simulink model "MCLV2_dsPIC33EP256MC506_externalOpAmp_DataLog"  (Simulink 9.2)
settings: Solver=FixedStepDiscrete  StartTime=0.0  StopTime=inf  FixedStep=.00005  RelTol=1e-3  EnableMultiTasking=on
undefined symbols (not defined in the file or in its folder): A4, A8, B5, B6, C10, C5, C6, D5, DiscIntNeverNeededParam, F0, F1, Max, ms, P20, P24, P53, P54, P97, Pin, PWMmax, Resol, us
libraries: MCHP_Blockset x19, simulink x16, simulink_need_slupdate x1
(part 2 of 2)

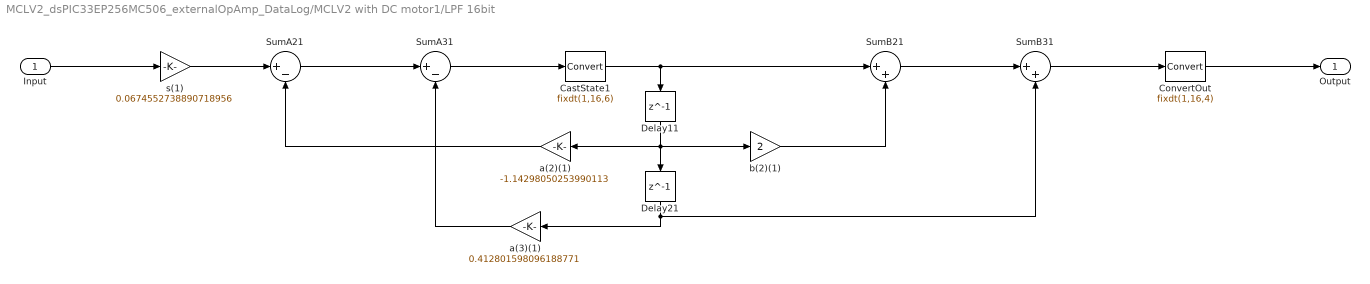
== system MCLV2_dsPIC33EP256MC506_externalOpAmp_DataLog/MCLV2 with DC motor1/LPF 16bit   ==
  Input : Inport
  CastState1 : DataTypeConversion  OutDataTypeStr=fixdt(1,16,6)
  ConvertOut : DataTypeConversion  OutDataTypeStr=fixdt(1,16,4)
  Delay11 : Delay  DelayLength=1  InitialCondition=0
  Delay21 : Delay  DelayLength=1  InitialCondition=0
  SumA21 : Sum  Inputs=|+-  AccumDataTypeStr=fixdt(1,16,6)  OutDataTypeStr=fixdt(1,16,6)
  SumA31 : Sum  Inputs=|+-  AccumDataTypeStr=fixdt(1,16,6)  OutDataTypeStr=fixdt(1,16,6)
  SumB21 : Sum  Inputs=|++  AccumDataTypeStr=fixdt(1,16,5)  OutDataTypeStr=fixdt(1,16,5)
  SumB31 : Sum  Inputs=|++  AccumDataTypeStr=fixdt(1,16,4)  OutDataTypeStr=fixdt(1,16,4)
  a(2)(1) : Gain  Gain=-1.14298050253990113  ParamDataTypeStr=fixdt(1,16,14)  OutDataTypeStr=fixdt(1,16,6)
  a(3)(1) : Gain  Gain=0.412801598096188771  ParamDataTypeStr=fixdt(0,16,17)  OutDataTypeStr=fixdt(1,16,8)
  b(2)(1) : Gain  Gain=2  ParamDataTypeStr=fixdt(0,16,14)  OutDataTypeStr=fixdt(1,16,5)
  s(1) : Gain  Gain=0.0674552738890718956  ParamDataTypeStr=fixdt(0,16,19)  OutDataTypeStr=fixdt(1,16,8)
  Output : Outport
  wires:
  s(1)/1 -> SumA21/1
  SumA21/1 -> SumA31/1
  SumA31/1 -> CastState1/1
  CastState1/1 -> SumB21/1, Delay11/1
  SumB21/1 -> SumB31/1
  SumB31/1 -> ConvertOut/1
  a(2)(1)/1 -> SumA21/2
  Delay11/1 -> a(2)(1)/1, b(2)(1)/1, Delay21/1
  b(2)(1)/1 -> SumB21/2
  a(3)(1)/1 -> SumA31/2
  Delay21/1 -> a(3)(1)/1, SumB31/2
  ConvertOut/1 -> Output/1
  Input/1 -> s(1)/1

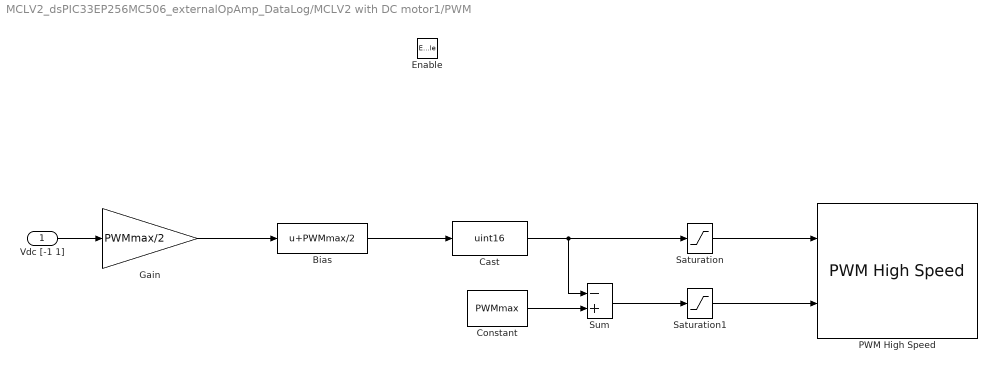
== system MCLV2_dsPIC33EP256MC506_externalOpAmp_DataLog/MCLV2 with DC motor1/PWM ==
  Vdc [-1 1] : Inport
  Enable : EnablePort
  Bias : Bias  Bias=PWMmax/2
  Cast : DataTypeConversion  OutDataTypeStr=uint16
  Constant : Constant  Value=PWMmax  OutDataTypeStr=uint16
  Gain : Gain  Gain=PWMmax/2  OutDataTypeStr=fixdt(1,32,1)
  PWM High Speed : MCHP_Blockset/PWM IO/PWM High Speed  pop1=[1]  chk1="[1  1  1  0  0]"  chkHL1="[1  1  0  1  1  1  1  1 ; 1  1  0  1  1  1  1  1]"  maxP1={ '50e-6','0.001','0.001','0.001','0.001','0.001','0.001','0.001';'0.001','0.001','1e-06','0.001','0.001','0.001','0.001','0.001'}  InitP2={ '50e-6','.001','0.001','0.001','0.001','0.001','0.001','0.001';'0.001','0.001','0.001','0.001','0.001','0.001','0.001','0.001'}  chkP2="[0  1  0  1  1  1  1  1 ; 1  0  0  1  1  1  1  1]"  InitDC={ '50','50','50','50','50','50','50','50';'0.001','0.001','0.001','50','50','50','50','50'}  chkDC="[1  1  1  1  1  1  1  1 ; 0  0  0  1  1  1  1  1]"  InitPh={ '0','0','0','0.001','0.001','0.001','0.001','0.001';'0','0','0','0.001','0.001','0.001','0.001','0.001'}  chkPh="[0  0  0  1  1  1  1  1 ; 0  0  0  1  1  1  1  1]"  edSEvTrigx={ '120e-9','-1','-1','-1','-1','-1','-1','-1'}  chkSEvTrigx="[0  1  1  1  1  1  1  1]"  popFlt="[2  2  1  1  1  1  1  1]"  popFltPin="[20  20  20   4   4   4   4   4]"  popFltPinRp="[1  1  1  1  1  1  1]"  popFltActivH="[2  2  1  1  1  1  1  1]"  popFltForceH="[2  2  2  2  2  2  2  2]"  popFltForceL="[1  1  1  1  1  1  1  1]"  chkFltBlkOut="[0  0  0  0  0  0  0  0]"  popIndepFaultMode="[1  1  1  1  1  1  1  1]"  popCurEnabled="[1  1  1  1  1  1  1  1]"  popCurPin="[4  31   4   4   4   4   4   4]"  popCurActiveH="[1  1  1  1  1  1  1  1]"  popCurForceH="[2  1  2  1  1  1  1  1]"  popCurForceL="[2  1  2  1  1  1  1  1]"  ChkCurBlkOut="[0  0  0  0  0  0  0  0]"  ChkCurBlkOutTime="[0  0  1  0  0  0  0  0]"  popBLANKSEL="[1  1  1  1  1  1  1  1]"  popBPHHBPHL="[1  1  1  1  1  1  1  1]"  popBPLHBPLL="[1  1  1  1  1  1  1  1]"  popFLTLEBEN_CLLEBEN="[1  1  1  1  1  1  1  1]"  popPHR_PHF="[2  1  1  1  1  1  1  1]"  popPLR_PLF="[3  1  1  1  1  1  1  1]"  edLEB={ '100e-9','50e-9','150e-9','50e-9','50e-9','50e-9','50e-9','50e-9'}  popDT="[1  1  1  3  3  3  3  3]"  edDTRx={ '0.02','1e-05','0.001','1e-05','1e-05','1e-05','1e-05','1e-05'}  edAltDTRx={ '0.5e-6','0.5e-6','Tm','1e-05','1e-05','1e-05','1e-05','1e-05'}  S_INPUT="[5  5  5]"  S_INPUT_Size="[1  1  1]"  S_OUTPUT=[]  S_OUTPUT_Size=[]  S_DWORK_Type=[]  S_DWORK_Size=[]  ADC_VARTRIG={PWM Primary Special Event Trigger;6}  SampleTime=-1  ORDERING=None  MCHP_PORT={PWM1 Fault}{FLT32}4:0:B4;{PWM2 Fault}{FLT32}4:0:B4;{PWM1H}{PWM1H}4:4:B14;{PWM1L}{PWM1L}4:4:B15;{PWM2H}{PWM2H}4:4:B12;{PWM2L}{PWM2L}4:4:B13;  MCHP_MASTERLINK=MCLV2_dsPIC33EP256MC506_externalOpAmp_DataLog/Microchip Master  MCHP_VERSION=v3.39
      settings: SourceProductName=MPLAB Device Blocks for Simulink
  Saturation : Saturate  UpperLimit=PWMmax - (1e-6/50e-6)*PWMmax  LowerLimit=round( (0.5e-6/50e-6) *PWMmax )
  Saturation1 : Saturate  UpperLimit=PWMmax  LowerLimit=round( (0.5e-6/50e-6) *PWMmax )
  Sum : Sum  Inputs=-+  OutDataTypeStr=Inherit: Same as first input
  wires:
  Gain/1 -> Bias/1
  Cast/1 -> Sum/1, Saturation/1
  Saturation/1 -> PWM High Speed/1
  Sum/1 -> Saturation1/1
  Bias/1 -> Cast/1
  Saturation1/1 -> PWM High Speed/2
  Vdc [-1 1]/1 -> Gain/1
  Constant/1 -> Sum/2

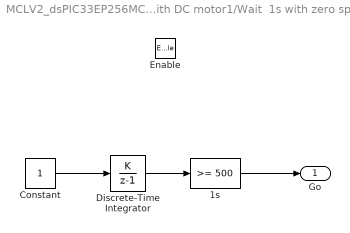
== system MCLV2_dsPIC33EP256MC506_externalOpAmp_DataLog/MCLV2 with DC motor1/Wait  1s with zero speed ==
  Enable : EnablePort
  "1s " : simulink/Logic and Bit Operations/Compare To Constant  relop=>=  const=500  OutDataTypeStr=boolean
  Constant : Constant  OutDataTypeStr=Inherit: Inherit via back propagation
  Discrete-Time Integrator : DiscreteIntegrator  IntegratorMethod=Accumulation: Forward Euler  gainval=1  SampleTime=-1  OutDataTypeStr=uint16  SaturateOnIntegerOverflow=on  ICPrevOutput=DiscIntNeverNeededParam  ICPrevScaledInput=DiscIntNeverNeededParam
  Go : Outport  InitialOutput=0
  wires:
  "1s "/1 -> Go/1
  Constant/1 -> Discrete-Time Integrator/1
  Discrete-Time Integrator/1 -> "1s "/1

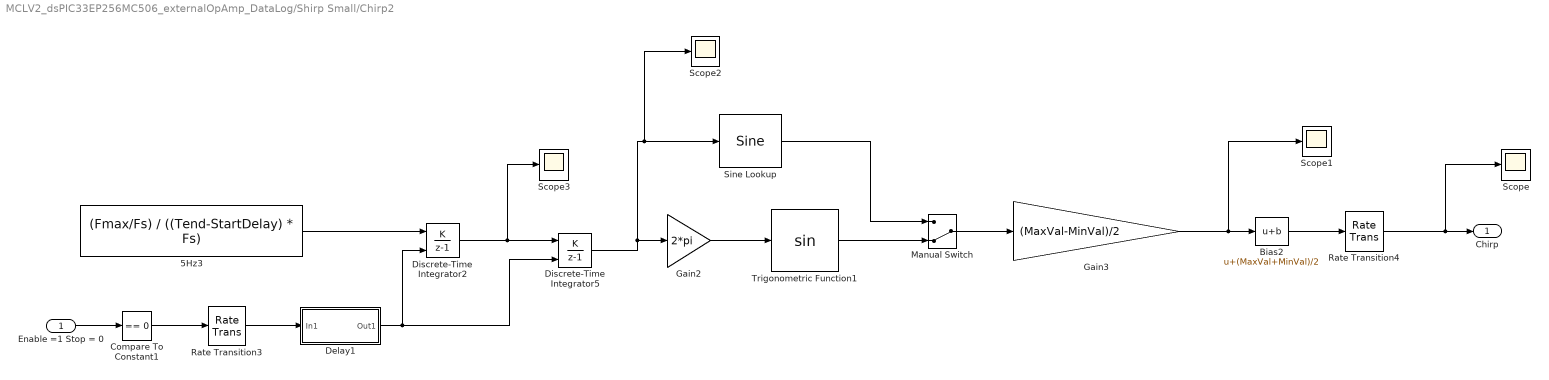
== system MCLV2_dsPIC33EP256MC506_externalOpAmp_DataLog/Shirp Small/Chirp2 ==
  Enable =1 Stop = 0 : Inport
  5Hz3 : Constant  Value=(Fmax/Fs) / ((Tend-StartDelay) * Fs)  VectorParams1D=off  OutMin=0  OutMax=Fmax/Fs  OutDataTypeStr=fixdt(0,32)  SampleTime=1/Fs
  Bias2 : Bias  Bias=(MaxVal+MinVal)/2
  Compare To Constant1 : simulink/Logic and Bit Operations/Compare To Constant  relop===  const=0  OutDataTypeStr=boolean
  Delay1 : Subsystem
  Discrete-Time Integrator2 : DiscreteIntegrator  IntegratorMethod=Accumulation: Forward Euler  gainval=1  ExternalReset=level  SampleTime=1/Fs  OutMax=Fmax/Fs  OutDataTypeStr=fixdt(0,32)  ICPrevOutput=DiscIntNeverNeededParam  ICPrevScaledInput=DiscIntNeverNeededParam
      settings: LockScale=on
  Discrete-Time Integrator5 : DiscreteIntegrator  IntegratorMethod=Accumulation: Forward Euler  gainval=1  ExternalReset=level  SampleTime=1/Fs  OutDataTypeStr=fixdt(0,16,16)  ICPrevOutput=DiscIntNeverNeededParam  ICPrevScaledInput=DiscIntNeverNeededParam
      settings: LockScale=on
  Gain2 : Gain  Gain=2*pi  OutDataTypeStr=fixdt(0,16,13)
  Gain3 : Gain  Gain=(MaxVal-MinVal)/2  OutMin=[MinVal]  OutMax=[MaxVal]  OutDataTypeStr=fixdt(1,16)
  Manual Switch : ManualSwitch  CurrentSetting=0
  Rate Transition3 : RateTransition  Deterministic=off
  Rate Transition4 : RateTransition  Deterministic=off
  Scope{,1..3} (4 alike) : Scope
  Sine Lookup : simulink/Lookup Tables/Sine  Formula=sin(2*pi*u)  NumDataPoints=(2^10)+1  OutputWordLength=16  InternalRulePriority=Speed
      settings: SourceProductName=Simulink
  Trigonometric Function1 : Trigonometry  ApproximationMethod=CORDIC
  Chirp : Outport
  wires:
  Enable =1 Stop = 0/1 -> Compare To Constant1/1
  Discrete-Time Integrator2/1 -> Scope3/1, Discrete-Time Integrator5/1
  5Hz3/1 -> Discrete-Time Integrator2/1
  Discrete-Time Integrator5/1 -> Scope2/1, Sine Lookup/1, Gain2/1
  Compare To Constant1/1 -> Rate Transition3/1
  Rate Transition3/1 -> Delay1/1(In1)
  Delay1/1(Out1) -> Discrete-Time Integrator5/2, Discrete-Time Integrator2/2
  Gain2/1 -> Trigonometric Function1/1
  Gain3/1 -> Scope1/1, Bias2/1
  Bias2/1 -> Rate Transition4/1
  Rate Transition4/1 -> Scope/1, Chirp/1
  Trigonometric Function1/1 -> Manual Switch/2
  Manual Switch/1 -> Gain3/1
  Sine Lookup/1 -> Manual Switch/1

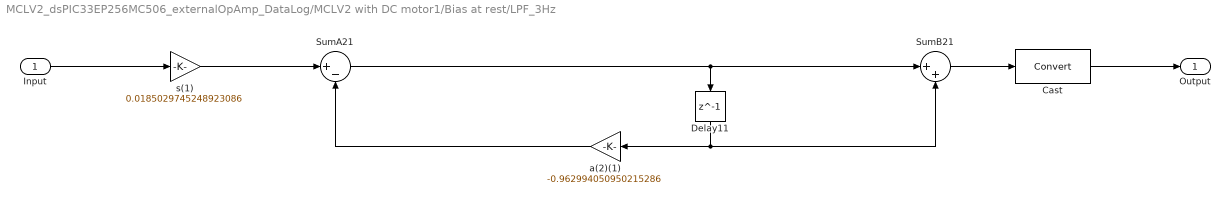
== system MCLV2_dsPIC33EP256MC506_externalOpAmp_DataLog/MCLV2 with DC motor1/Bias at rest/LPF_3Hz ==
  Input : Inport
  Cast : DataTypeConversion
  Delay11 : Delay  DelayLength=1  InitialCondition=0
  SumA21 : Sum  Inputs=|+-  RndMeth=Convergent  SaturateOnIntegerOverflow=on  OutDataTypeStr=Inherit: Same as first input
  SumB21 : Sum  Inputs=|++  RndMeth=Simplest  SaturateOnIntegerOverflow=on  OutDataTypeStr=Inherit: Same as first input
  a(2)(1) : Gain  Gain=-0.962994050950215286  ParamDataTypeStr=fixdt(1,16,14)  RndMeth=Simplest  OutDataTypeStr=Inherit: Same as input
  s(1) : Gain  Gain=0.0185029745248923086  ParamDataTypeStr=fixdt(1,16,20)  OutDataTypeStr=fixdt(1,16,16)  RndMeth=Convergent  SaturateOnIntegerOverflow=on
  Output : Outport
  wires:
  s(1)/1 -> SumA21/1
  SumA21/1 -> SumB21/1, Delay11/1
  a(2)(1)/1 -> SumA21/2
  Delay11/1 -> a(2)(1)/1, SumB21/2
  SumB21/1 -> Cast/1
  Input/1 -> s(1)/1
  Cast/1 -> Output/1

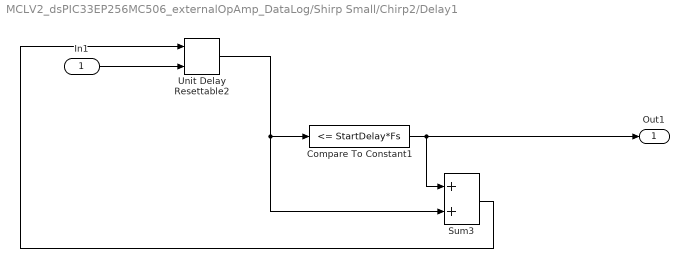
== system MCLV2_dsPIC33EP256MC506_externalOpAmp_DataLog/Shirp Small/Chirp2/Delay1 ==
  In1 : Inport
  Compare To Constant1 : simulink/Logic and Bit Operations/Compare To Constant  relop=<=  const=StartDelay*Fs  OutDataTypeStr=boolean
  Sum3 : Sum  AccumDataTypeStr=uint16  OutDataTypeStr=Inherit: Same as accumulator
  Unit Delay Resettable2 : simulink_need_slupdate/Unit Delay Resettable  vinit=1  tsamp=inv(Fs)
      settings: SourceProductName=Simulink  SourceProductBaseCode=SL
  Out1 : Outport
  wires:
  Unit Delay Resettable2/1 -> Sum3/2, Compare To Constant1/1
  In1/1 -> Unit Delay Resettable2/2
  Sum3/1 -> Unit Delay Resettable2/1
  Compare To Constant1/1 -> Out1/1, Sum3/1
